simulink model "SystemCtrl"  (R2018b)
settings: Solver=VariableStepAuto  StartTime=0.0  StopTime=10.0  RelTol=1e-3
values from neighbouring files (symbols this model uses):
  A = [a Znm; -c Zmm]    [LQG_example.m]    (also in Linearize.m = double(subs(A_mat,[alpha,beta,gamma,F_f,F_b],[x_s(1:3),u_s(1)
  B = [b;-d]    [LQG_example.m]    (also in Linearize.m = double(subs(B_mat,[alpha,beta,gamma],x_s(1:3))))
  C = [eye(3),zeros(3,3)]    [Linearize.m]
  D = zeros(3,2)    [Linearize.m]
settings Model: Creator=boateng  LastModifiedBy=boateng

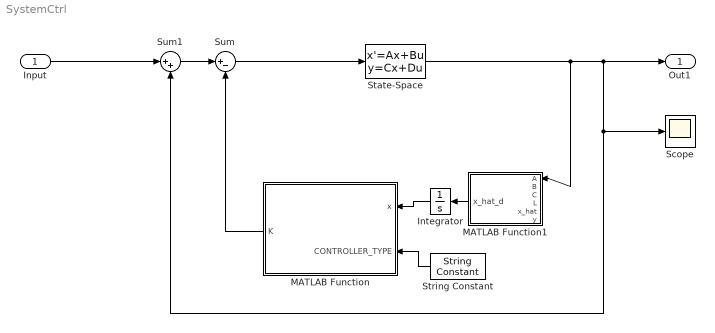
== system SystemCtrl ==
  Input : Inport
  Integrator : Integrator
  MATLAB Function : MATLAB Function  TreatAsAtomicUnit=on
  MATLAB Function1 : MATLAB Function  TreatAsAtomicUnit=on
  Scope : Scope
  State-Space : StateSpace  A=A  B=B  C=C  D=D  InitialCondition=0
  String Constant : StringConstant  String="\"LQR\""
  Sum : Sum  Inputs=|+-
  Sum1 : Sum  Inputs=|++
  Out1 : Outport
  wires:
  MATLAB Function/1(K) -> Sum/2
  Sum/1 -> State-Space/1
  String Constant/1 -> MATLAB Function/2(CONTROLLER_TYPE)
  Integrator/1 -> MATLAB Function/1(x)
  MATLAB Function1/1(x_hat_d) -> Integrator/1
  Sum1/1 -> Sum/1
  Input/1 -> Sum1/1
  State-Space/1 -> MATLAB Function1/1(A), Out1/1, Scope/1, Sum1/2

== matlab function SystemCtrl/MATLAB Function1 ==
  data: A input; x_hat_d output; B input; C input; L input; x_hat input; y input
function x_hat_d = state_observer(A,B,C, L, x_hat, y)

x_hat_d = A*x_hat+B*u+L*(y-C*x_hat);

== matlab function SystemCtrl/MATLAB Function ==
  data: x input; K output; CONTROLLER_TYPE input
function K  = lqr_controller(x, CONTROLLER_TYPE)
    
    run('Linearize.m')

    p=size(3,1);                    % no. of outputs (y)
    [n,z]=size(B);                  % no. of states nd inputs (u)(6,2)
    F=zeros(n,z); 
    T=zeros(z,z); 
    W=zeros(n,n); 
    H=zeros(z,n);
    % 1) Design a state feedback controller
    %A_aug=[A F; -C T]; 
    %B_aug=[B;-D];                   % augment plant with integrators
    Q_I=eye(9);             % weight on integrated error
    Q=eye(n);
    R=eye(z);   
    
    %to compare both controller build switch
    if strcmp(CONTROLLER_TYPE, 'LQR')
        [Kr,P,EW]=lqr(A,B,Q,R);
        K=Kr
    else 
        [Kr_I,P_I,EW_I] = lqi(plant,Q_I,R,0);
        K= Kr_I
    end
% input weight
%     [Kr,P,EW]=lqr(A,B,Q,R);
%     [Kr_I,P_I,EW_I] = lqi(plant,Q_I,R,0);
    
end
